simulink model "Sim_OutputLQR"  (R2017b)
settings: Solver=FixedStepAuto  StartTime=0.0  StopTime=20  FixedStep=0.001  RelTol=1e-3
values from neighbouring files (symbols this model uses):
  A = [0 1;0 0]    [LQRTest.m]    (also in OptimalOutputFeedback.m; Prob2_Hw3.m; Prob3.m = [Lp 0 Ldela; Prob3_LQR.m = [Lp 0 Ldela)
  B = [0 1]'    [LQRTest.m]    (also in OptimalOutputFeedback.m; Prob2_Hw3.m; Prob3.m = [0 0 1/tau]'; Prob3_LQR.m = [0 0 1/tau]')
  C = [1 1]    [LQRTest.m]    (also in OptimalOutputFeedback.m; Prob2_Hw3.m; Prob3.m = [0 1 1]; Prob3_LQR.m = [0 1 1])
  K = K_new(end)    [LQRTest.m]    (also in OptimalOutputFeedback.m = K_k(end); Prob2_Hw3.m = K(end); Prob3_LQR.m = k; Prob4.m = [K11,K12)
  x0 = [1 1]'    [LQRTest.m]    (also in OptimalOutputFeedback.m = [1 0]'; Prob2_Hw3.m = [0 1]'; Prob3.m = [1 0.1 0]'; Prob3_LQR.m = [1 0.1 0]')
settings Model: Creator=Daslab  LastModifiedBy=thapa

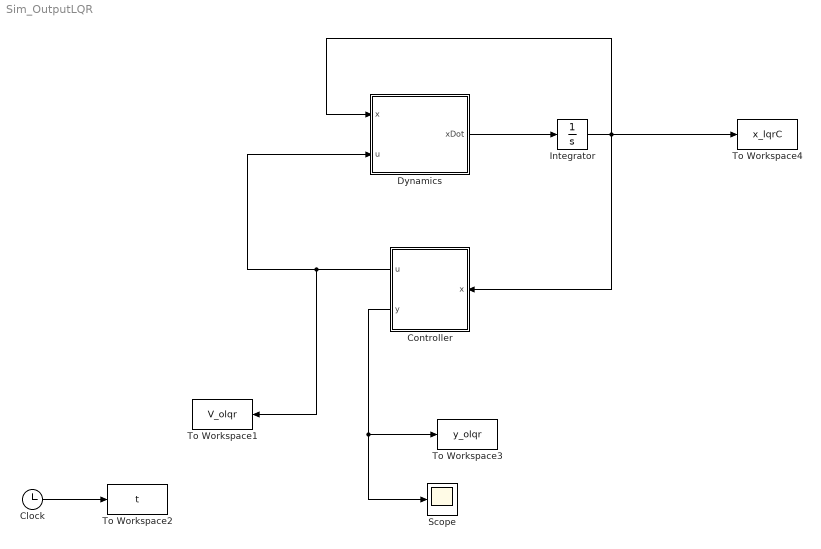
== system Sim_OutputLQR ==
  Clock : Clock
  Controller : MATLAB Function  TreatAsAtomicUnit=on
  Dynamics : MATLAB Function  TreatAsAtomicUnit=on
  Integrator : Integrator  InitialCondition=x0
  Scope : Scope
  To Workspace1 : ToWorkspace  VariableName=V_olqr  SampleTime=-1
      settings: Save2DSignal=2-D array (concatenate along first dimension)
  To Workspace2 : ToWorkspace  VariableName=t  SampleTime=-1
      settings: Save2DSignal=2-D array (concatenate along first dimension)
  To Workspace3 : ToWorkspace  VariableName=y_olqr  SampleTime=-1
      settings: Save2DSignal=2-D array (concatenate along first dimension)
  To Workspace4 : ToWorkspace  VariableName=x_lqrC  SampleTime=-1
      settings: Save2DSignal=2-D array (concatenate along first dimension)
  wires:
  Dynamics/1(xDot) -> Integrator/1
  Integrator/1 -> Controller/1(x), Dynamics/1(x), To Workspace4/1
  Controller/1(u) -> To Workspace1/1, Dynamics/2(u)
  Clock/1 -> To Workspace2/1
  Controller/2(y) -> To Workspace3/1, Scope/1

== matlab function Sim_OutputLQR/Controller ==
  data: x input; u output; y output; C parameter; K parameter
function [u,y] = Controller(x,C, K)

y = C*x;
u = -K*y;

== matlab function Sim_OutputLQR/Dynamics ==
  data: x input; u input; xDot output; B parameter; A parameter
function xDot = Dynamics(x,u, B, A)

xDot = A*x + B*u;
